simulink model "testMatlabFunction"  (R2015a)
settings: Solver=ode45  StartTime=0.0  StopTime=100  RelTol=1e-3
settings Model: Creator=shawn  LastModifiedBy=shawn

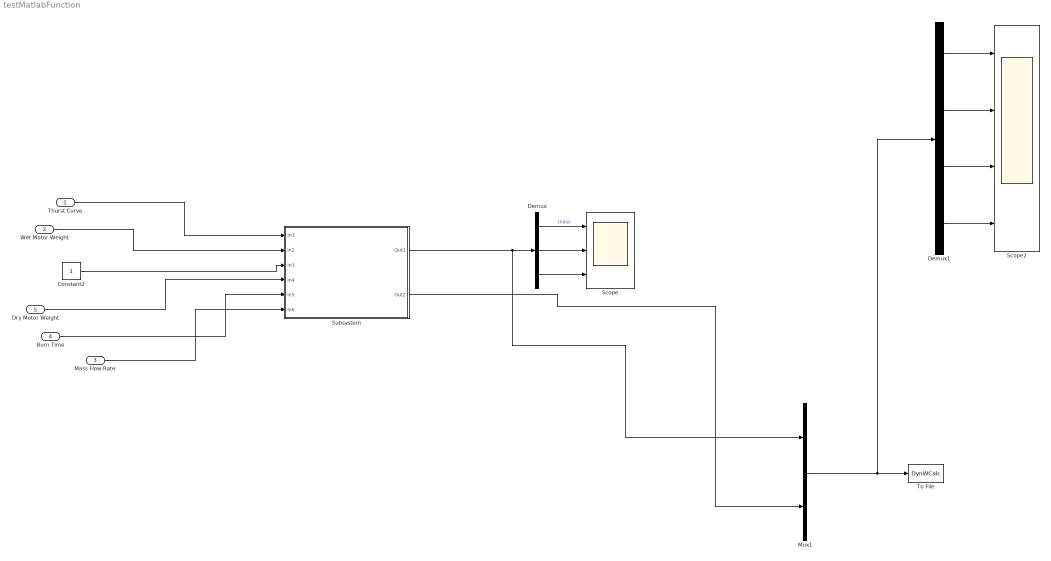
== system testMatlabFunction ==
  Thurst Curve : Inport
  Wet Motor Weight : Inport  Port=2
  Mass Flow Rate : Inport  Port=3
  Burn Time : Inport  Port=4
  Dry Motor Weight : Inport  Port=5
  Constant2 : Constant
  Demux : Demux  Outputs=[1 1 1]
  Demux1 : Demux
  Mux1 : Mux  Inputs=2
  Scope : Scope  NumInputPorts=3
      settings: YMin=-5~-5~-5  YMax=5~5~5
  Scope2 : Scope  NumInputPorts=4
      settings: YMin=-5~-5~-5~-5  YMax=5~5~5~5  SaveName=ScopeData2
  Subsystem : Subsystem
  To File : ToFile  Filename=DynWCalc
  wires:
  Demux/1 -> Scope/1  "mass"
  Demux/2 -> Scope/2
  Demux/3 -> Scope/3
  Demux1/3 -> Scope2/3
  Demux1/4 -> Scope2/4
  Demux1/2 -> Scope2/2
  Demux1/1 -> Scope2/1
  Mux1/1 -> Demux1/1, To File/1
  Subsystem/1(Out1) -> Mux1/1, Demux/1
  Thurst Curve/1 -> Subsystem/1(In1)
  Wet Motor Weight/1 -> Subsystem/2(In2)
  Constant2/1 -> Subsystem/3(In3)
  Dry Motor Weight/1 -> Subsystem/4(In4)
  Burn Time/1 -> Subsystem/5(In5)
  Mass Flow Rate/1 -> Subsystem/6(In6)
  Subsystem/2(Out2) -> Mux1/2

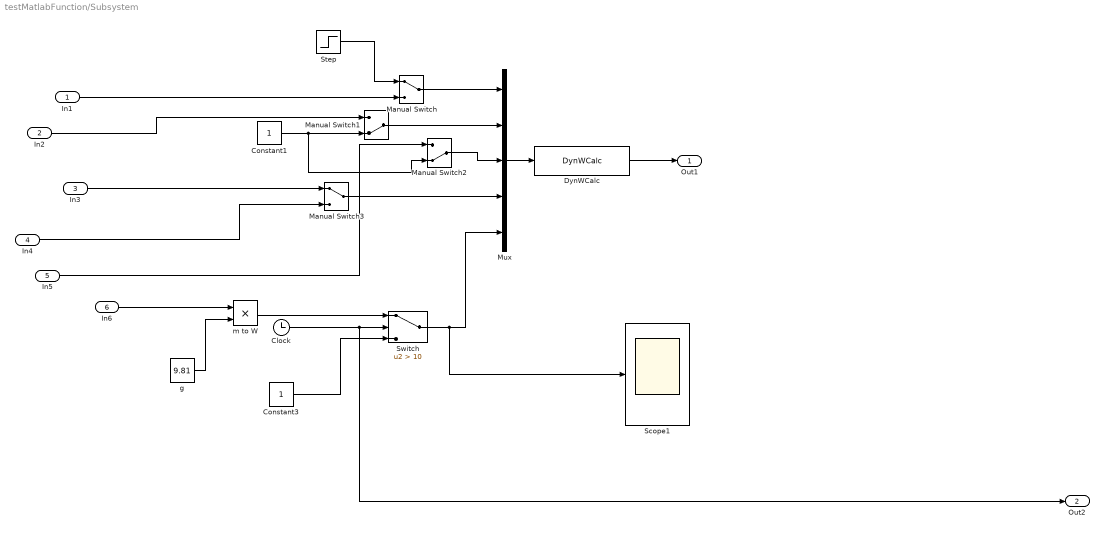
== system testMatlabFunction/Subsystem ==
  In1 : Inport
  In2 : Inport  Port=2
  In3 : Inport  Port=3
  In4 : Inport  Port=4
  In5 : Inport  Port=5
  In6 : Inport  Port=6
  Clock : Clock
  Constant1 : Constant
  Constant3 : Constant
  DynWCalc : MATLABFcn  MATLABFcn=DynWCalc
      mask Display: disp('DynWCalc')
  Manual Switch : ManualSwitch
  Manual Switch1 : ManualSwitch  CurrentSetting=0
  Manual Switch2 : ManualSwitch  CurrentSetting=0
  Manual Switch3 : ManualSwitch
  Mux : Mux  Inputs=5
  Scope1 : Scope
  Step : Step  SampleTime=0
  Switch : Switch  Criteria=u2 > Threshold  Threshold=10
  g : Constant  Value=9.81
  m to W : Product
  Out1 : Outport
  Out2 : Outport  Port=2
  wires:
  Step/1 -> Manual Switch/1
  DynWCalc/1 -> Out1/1
  Manual Switch2/1 -> Mux/3
  Constant1/1 -> Manual Switch2/2, Manual Switch1/2
  Manual Switch3/1 -> Mux/4
  In3/1 -> Manual Switch3/1
  In5/1 -> Manual Switch2/1
  In1/1 -> Manual Switch/2
  In6/1 -> m to W/1
  Manual Switch/1 -> Mux/1
  g/1 -> m to W/2
  Switch/1 -> Scope1/1, Mux/5
  Mux/1 -> DynWCalc/1
  In4/1 -> Manual Switch3/2
  m to W/1 -> Switch/1
  In2/1 -> Manual Switch1/1
  Constant3/1 -> Switch/3
  Clock/1 -> Out2/1, Switch/2
  Manual Switch1/1 -> Mux/2
